simulink subsystem "SubSystemExtruder"  (R2020b)
settings: Solver=VariableStepAuto  StartTime=0.0  StopTime=10.0  RelTol=1e-3
libraries: simulink x2
settings Model: Creator=kaebi  LastModifiedBy=kaebi

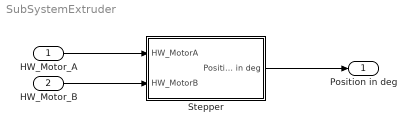
== system SubSystemExtruder ==
  HW_Motor_A : Inport
  HW_Motor_B : Inport  Port=2
  Stepper : Subsystem
  Position in deg : Outport
  wires:
  HW_Motor_A/1 -> Stepper/1(HW_MotorA)
  HW_Motor_B/1 -> Stepper/2(HW_MotorB)
  Stepper/1(Position in deg) -> Position in deg/1

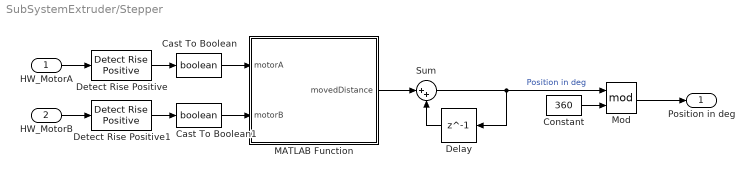
== system SubSystemExtruder/Stepper ==
  HW_MotorA : Inport
  HW_MotorB : Inport  Port=2
  Cast To Boolean : DataTypeConversion  OutDataTypeStr=boolean
  Cast To Boolean1 : DataTypeConversion  OutDataTypeStr=boolean
  Constant : Constant  Value=360
  Delay : Delay  DelayLength=1
  Detect Rise Positive : simulink/Logic and Bit Operations/Detect Rise Positive  vinit=0  OutDataTypeStr=boolean
  Detect Rise Positive1 : simulink/Logic and Bit Operations/Detect Rise Positive  vinit=0  OutDataTypeStr=boolean
  MATLAB Function : MATLAB Function  TreatAsAtomicUnit=on
  Mod : Math  Operator=mod  SaturateOnIntegerOverflow=on
  Sum : Sum  Inputs=|++
  Position in deg : Outport
  wires:
  Delay/1 -> Sum/2
  HW_MotorB/1 -> Detect Rise Positive1/1
  Cast To Boolean1/1 -> MATLAB Function/2(motorB)
  Cast To Boolean/1 -> MATLAB Function/1(motorA)
  MATLAB Function/1(movedDistance) -> Sum/1
  HW_MotorA/1 -> Detect Rise Positive/1
  Sum/1 -> Mod/1, Delay/1  "Position in deg"
  Detect Rise Positive/1 -> Cast To Boolean/1
  Constant/1 -> Mod/2
  Detect Rise Positive1/1 -> Cast To Boolean1/1
  Mod/1 -> Position in deg/1

== matlab function SubSystemExtruder/Stepper/MATLAB Function ==
  settings: updateMethod=DISCRETE
  data: motorA input; movedDistance output; motorB input
function movedDistance  = fcn(motorA, motorB)
    persistent isOnA;
    
    if isempty(isOnA)
        isOnA = false;
    end

    degPerStep = 360/200;
    movedDistance = 0;
    
    if (motorA == true && isOnA == false)
        movedDistance = degPerStep;
        isOnA = true;
    elseif (motorB == true && isOnA == true)
        movedDistance = degPerStep;
        isOnA = false;
    end
    
end
